simulink model "non_linear_model"  (R2021a)
settings: Solver=FixedStepAuto  StartTime=0.0  StopTime=T  FixedStep=sim_step  RelTol=1e-3
values from neighbouring files (symbols this model uses):
  g = 9.81    [model_structure_linera.m]    (also in model_structure_non_linera.m; non_linear.m; pedulum_simulation.m; real_pend_sim.m)
  l = 1    [non_linear.m]    (also in pedulum_simulation.m = 0.5; real_pend_sim.m = 0.5)
  M = 0.5723    [model_structure_linera.m]    (also in model_structure_non_linera.m; non_linear.m = 1; pedulum_simulation.m; real_pend_sim.m)
  m = 0.12    [model_structure_linera.m]    (also in model_structure_non_linera.m; non_linear.m = 0.5; pedulum_simulation.m; real_pend_sim.m)
libraries: slident x1
settings Model: Creator=kpiek  LastModifiedBy=kpiek
settings DebuggingCC: AlgebraicLoopMsg=none

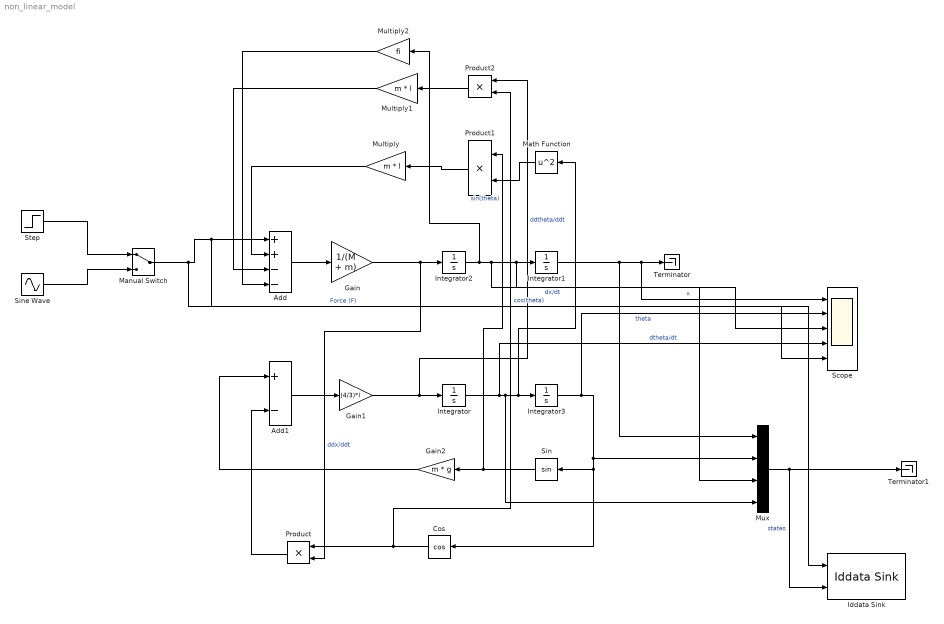
== system non_linear_model ==
  Add : Sum  Inputs=++--
  Add1 : Sum  Inputs=+-
  Cos : Trigonometry  Operator=cos
  Gain : Gain  Gain=1/(M + m)
  Gain1 : Gain  Gain=(4/3)*l
  Gain2 : Gain  Gain=m * g
  Iddata Sink : slident/Iddata Sink  datasetname=data  Ts=0.1  isu=on  isy=on
      settings: SourceProductBaseCode=ID
  Integrator : Integrator
  Integrator1 : Integrator
  Integrator2 : Integrator
  Integrator3 : Integrator  InitialCondition=pi
  Manual Switch : ManualSwitch
  Math Function : Math  Operator=square  SaturateOnIntegerOverflow=on
  Multiply : Gain  Gain=m * l
  Multiply1 : Gain  Gain=m * l
  Multiply2 : Gain  Gain=fi
  Mux : Mux
  Product : Product
  Product1 : Product
  Product2 : Product
  Scope : Scope  NumInputPorts=5
  Sin : Trigonometry
  Sine Wave : Sin  SampleTime=0
  Step : Step  SampleTime=0
  Terminator : Terminator
  Terminator1 : Terminator
  wires:
  Add/1 -> Gain/1
  Gain/1 -> Product/2, Integrator2/1  "ddx/ddt"
  Add1/1 -> Gain1/1
  Gain1/1 -> Product2/1, Integrator/1  "ddtheta/ddt"
  Integrator/1 -> Scope/4, Mux/4, Math Function/1, Integrator3/1  "dtheta/dt"
  Integrator2/1 -> Multiply2/1, Scope/3, Mux/3, Integrator1/1  "dx/dt"
  Integrator1/1 -> Mux/1, Scope/1, Terminator/1  "x"
  Integrator3/1 -> Scope/2, Mux/2, Cos/1, Sin/1  "theta"
  Sin/1 -> Product1/1, Gain2/1  "sin(theta)"
  Gain2/1 -> Add1/1
  Cos/1 -> Product2/2, Product/1  "cos(theta)"
  Product/1 -> Add1/2
  Product1/1 -> Multiply/1
  Math Function/1 -> Product1/2
  Multiply/1 -> Add/2
  Product2/1 -> Multiply1/1
  Multiply1/1 -> Add/3
  Multiply2/1 -> Add/4
  Step/1 -> Manual Switch/1
  Sine Wave/1 -> Manual Switch/2
  Manual Switch/1 -> Iddata Sink/1, Scope/5, Add/1  "Force (F)"
  Mux/1 -> Iddata Sink/2, Terminator1/1  "states"
